simulink model "plant2MRUEBF3_max12"  (R2023b)
settings: Solver=VariableStepAuto  StartTime=0.0  StopTime=7  RelTol=1e-3
model workspace (MATLAB code in the model file):
  | %% Paramètres du Système
  | % Masses
  | mw=0.06;
  | mb=0.894;
  | Ms=mb + 2*mw;
  | 
  | % Distances
  | rho=0.036;
  | l=0.165;
  | d=0.086; % distance A-C
  | 
  | % Electriques
  | L=2.3e-3;
  | R=2.2;
  | % r;
  | 
  | % Couples
  | k=0.347;
  | % alpha=33.5;
  | % beta=2.26e-2;
  | 
  | % Moments inertie A TROUVER
  | Iwy=1.6e-4;
  | Ipsi=3.12e-2;
  | 
  | % Constantes utilitaires
  | beta = (Ms + 2*Iwy/rho^2);
  | gamma = Ipsi + mb*d^2;
  | alpha = 2/rho;
  | eta = l/rho;
  | 
  | % Largeur SensorBar
  | dCLF = 0.09;
  | 
  | %% Trajectoire d'équilibre
  | % Mouvement Rectiligne Uniforme selon axe x du laboratoire.
  | % On néglige les perturbations sur les entrées et les mesures.
  | 
  | % Références
  | ur = 0.3; %m/s
  | psir = 0;
  | 
  | % On fait le changement right,left (r,l) -> sum,dif (s,d)
  | % Somme des tensions gauche et droite
  | % Le "s" signifie "sum", on trouvera aussi "d"
  | % pour "difference"
  | Usbar = 2*k/rho*ur; % should not be >12V
  | Udbar = 0;
  | 
  | Urbar = Usbar/2;
  | Ulbar = Usbar/2;
  | 
  | pbar = 0; % normally, should equals ubar*t,
  | % but is not in state function, so any value fits.
  | ubar = ur;
  | psibar = psir;
  | vbar = 0;
  | Isbar = 0;
  | Idbar = 0;
  | ybar = 0;
  | 
  | statebar = [pbar; ubar; psibar; vbar; Isbar; Idbar; ybar];
  | 
  | %% Sous-système Lent Somme
  | % On a négligé Is par perturbation
  | % Etat=[p; u], Entrée=[Us], Sortie mesurée=[phis]
  | 
  | Qs = k/beta/rho/R;
  | 
  | ASum = [0 1;
  |     0 Qs*(-2*k/rho)];
  | 
  | BSum = [0;
  |     Qs];
  | 
  | CSum = [alpha 0];
  | 
  | DSum = [0];
  | 
  | sysSum = augstate(ss(ASum,BSum,CSum,DSum)); % Ajout de l'état à la sortie
  | set(sysSum,'InputName',{'dUs'},'OutputName',{'dphis','dp','du'});
  | 
  | %% Sous-système Lent Différence
  | % On a négligé Id par perturbation
  | % Etat=[psi; v; y], Entrée=[Ud], Sortie mesurée=[phid; cLF]
  | 
  | b1 = 1/gamma*mb*d*ubar;
  | b2 = 1/gamma*l*k/2/rho/R;
  | 
  | ADif = [0 1 0;
  |     0 (b1 + b2*(-k*l/rho)) 0;
  |     ubar 0 0];
  | 
  | BDif = [0;
  |     b2;
  |     0];
  | 
  | CDif = [eta 0 0;
  |     0 0 1];
  | 
  | DDif = [0;
  |     0];
  | 
  | sysDif = augstate(ss(ADif,BDif,CDif,DDif)); % Ajout de l'état à la sortie
  | set(sysDif,'InputName',{'dUd'},'OutputName',{'dphid','dcLF','dpsi','dv', ...
  |     'dy'});
  | 
  | %% Contrôleurs
  | 
  | %% Modèle de commande somme
  | % réglage PD idéal
  | sumEig = sort(eig(ASum));
  | w0 = 1*abs(sumEig(1)); % accélération facteur 2000
  | xi = 1/sqrt(2);
  | % Gains
  | h1 = w0^2/Qs/alpha;
  | h2 = 1/alpha*(-2*xi*w0/Qs + 2*k/rho);
  | h3 = h1;
  | 
  | % PD approximé
  | Tds = h2/h1;
  | ns = 150; % à régler, augmente la sensibilité au bruit.
  | 
  | 
  | %% Modèle de commande diff
  | 
  | % réglage Contrôleur Idéal, PD sur phid, P sur cLF
  | sigma = 15; % à régler, réponse très lente.
  | % Gains
  | k1 = 1/b2/eta*sigma^2*sqrt(6);
  | k2 = 1/b2/eta*(-sigma*sqrt(6) - b1 + b2*k*l/rho);
  | k3 = k1;
  | k4 = sigma^3/ubar/b2;
  | k5 = k4;
  | difEigDesired = roots([1 sigma*sqrt(6) sigma^2*sqrt(6) sigma^3]);
  | 
  | % PD+D idéal
  | PDdif = [tf([-k2 k3],1) tf([k5],1) tf([k2 -k1],1) tf([-k4],1)];
  | 
  | % PD+P approximé
  | Tdd = k2/k1;
  | nd = 150;
  | 
  | Md = -nd;
  | Nd = [nd 0 -nd 0];
  | Pd = k1*Tdd*nd;
  | Qd = [k1*(1-Tdd*nd) k5 -k1*(1-Tdd*nd) -k5];
  | 
  | %% Etat initial perturbé pour test en poursuite
  | 
  | delta_y = 0.03;
  | delta_psi = pi/2;
  | statebar_perturb = [pbar; ubar; psibar; vbar; Isbar; Idbar; ybar + delta_y];
settings Model: Creator=Jules  LastModifiedBy=Jules

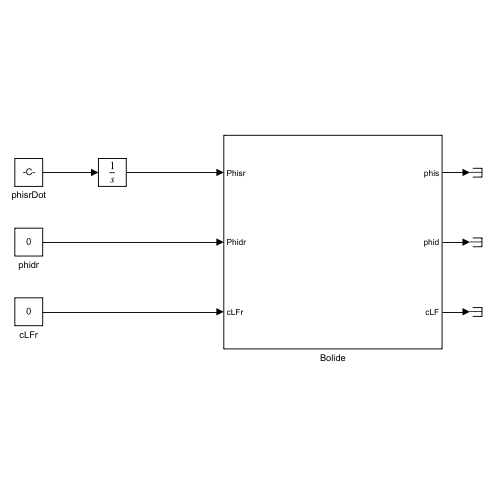
[thumbnail: Simulink's stored preview of the top-level diagram]
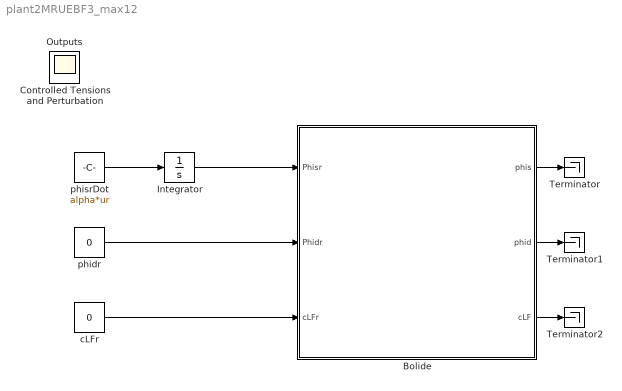
== system plant2MRUEBF3_max12 ==
  Bolide : Subsystem
  Integrator : Integrator
  Terminator : Terminator
  Terminator1 : Terminator
  Terminator2 : Terminator
  cLFr : Constant  Value=0
  phidr : Constant  Value=0
  phisrDot : Constant  Value=alpha*ur
  Controlled Tensions and Perturbation : Scope
  Outputs : Scope
  wires:
  Integrator/1 -> Bolide/1(Phisr)
  phisrDot/1 -> Integrator/1
  phidr/1 -> Bolide/2(Phidr)
  cLFr/1 -> Bolide/3(cLFr)
  Bolide/3(cLF) -> Terminator2/1
  Bolide/2(phid) -> Terminator1/1
  Bolide/1(phis) -> Terminator/1

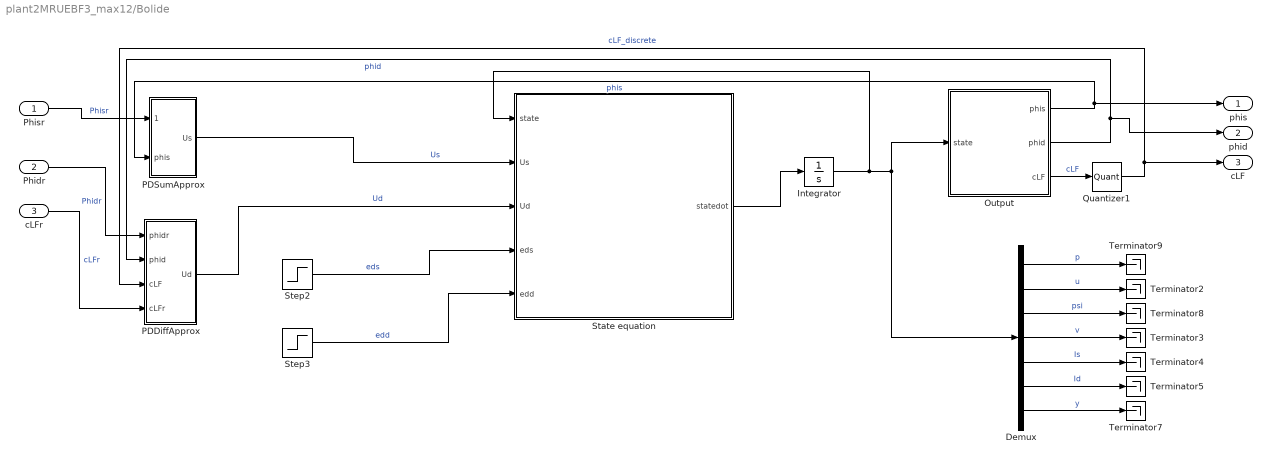
== system plant2MRUEBF3_max12/Bolide ==
  Phisr : Inport
  Phidr : Inport  Port=2
  cLFr : Inport  Port=3
  Demux : Demux  Outputs=7
  Integrator : Integrator  InitialCondition=statebar_perturb
  Output : MATLAB Function  TreatAsAtomicUnit=on
  PDDiffApprox : Subsystem
  PDSumApprox : Subsystem
  Quantizer1 : Quantizer  QuantizationInterval=dCLF/7
  State equation : MATLAB Function  TreatAsAtomicUnit=on
  Step2 : Step  Time=5  After=0  SampleTime=0
  Step3 : Step  Time=2  After=0  SampleTime=0
  Terminator{2..5,7..9} (7 alike) : Terminator
  phis : Outport
  phid : Outport  Port=2
  cLF : Outport  Port=3
  wires:
  Step3/1 -> State equation/5(edd)  "edd"
  State equation/1(statedot) -> Integrator/1
  Step2/1 -> State equation/4(eds)  "eds"
  Demux/1 -> Terminator9/1  "p"
  Demux/7 -> Terminator7/1  "y"
  Demux/2 -> Terminator2/1  "u"
  Demux/6 -> Terminator5/1  "Id"
  Demux/4 -> Terminator3/1  "v"
  Demux/5 -> Terminator4/1  "Is"
  Demux/3 -> Terminator8/1  "psi"
  PDDiffApprox/1(Ud) -> State equation/3(Ud)  "Ud"
  Integrator/1 -> Output/1(state), Demux/1, State equation/1(state)
  Output/1(phis) -> PDSumApprox/2(phis), phis/1  "phis"
  Output/2(phid) -> phid/1, PDDiffApprox/2(phid)  "phid"
  Quantizer1/1 -> PDDiffApprox/3(cLF), cLF/1  "cLF_discrete"
  Phisr/1 -> PDSumApprox/1(phisr)  "Phisr"
  PDSumApprox/1(Us) -> State equation/2(Us)  "Us"
  cLFr/1 -> PDDiffApprox/4(cLFr)  "cLFr"
  Phidr/1 -> PDDiffApprox/1(phidr)  "Phidr"
  Output/3(cLF) -> Quantizer1/1  "cLF"

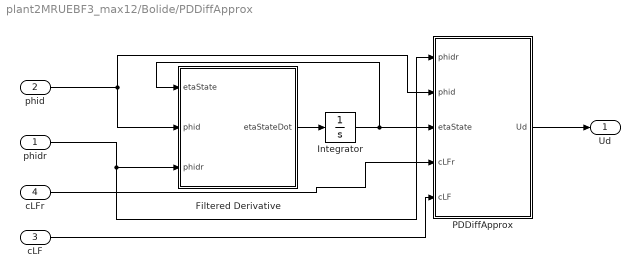
== system plant2MRUEBF3_max12/Bolide/PDDiffApprox ==
  phidr : Inport
  phid : Inport  Port=2
  cLF : Inport  Port=3
  cLFr : Inport  Port=4
  Filtered Derivative : MATLAB Function  TreatAsAtomicUnit=on
  Integrator : Integrator
  PDDiffApprox : MATLAB Function  TreatAsAtomicUnit=on
  Ud : Outport
  wires:
  phidr/1 -> PDDiffApprox/1(phidr), Filtered Derivative/3(phidr)
  phid/1 -> Filtered Derivative/2(phid), PDDiffApprox/2(phid)
  Filtered Derivative/1(etaStateDot) -> Integrator/1
  Integrator/1 -> Filtered Derivative/1(etaState), PDDiffApprox/3(etaState)
  PDDiffApprox/1(Ud) -> Ud/1
  cLF/1 -> PDDiffApprox/5(cLF)
  cLFr/1 -> PDDiffApprox/4(cLFr)

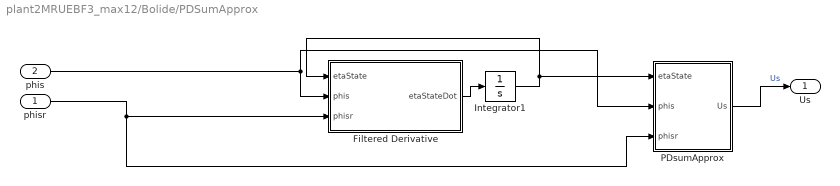
== system plant2MRUEBF3_max12/Bolide/PDSumApprox ==
  phisr : Inport
  phis : Inport  Port=2
  Filtered Derivative : MATLAB Function  TreatAsAtomicUnit=on
  Integrator1 : Integrator
  PDsumApprox : MATLAB Function  TreatAsAtomicUnit=on
  Us : Outport
  wires:
  Integrator1/1 -> Filtered Derivative/1(etaState), PDsumApprox/1(etaState)
  phis/1 -> Filtered Derivative/2(phis), PDsumApprox/2(phis)
  Filtered Derivative/1(etaStateDot) -> Integrator1/1
  phisr/1 -> PDsumApprox/3(phisr), Filtered Derivative/3(phisr)
  PDsumApprox/1(Us) -> Us/1  "Us"

== matlab function plant2MRUEBF3_max12/Bolide/PDSumApprox/Filtered Derivative ==
  data: etaState input; etaStateDot output; phis input; phisr input; ns parameter
function etaStateDot = fcn(etaState,phis,phisr,ns)
deltaPhisr = (phisr - phis);
etaStateDot = ns*(deltaPhisr - etaState);

== matlab function plant2MRUEBF3_max12/Bolide/State equation ==
  data: state input; statedot output; Us input; Ud input; eds input; edd input; beta parameter; gamma parameter; rho parameter; l parameter; d parameter; L parameter; R parameter; k parameter; mb parameter
function statedot = fcn(state, Us, Ud, eds, edd, beta, gamma, rho, l, d, L, R, k, mb)
% ed est l'entrée de perturbation, != d (distance AC)
% Model parameters defined in "Model Explorer/Matlab Code"

p = state(1); % intégrale temporelle de u, distance parcourue
u = state(2);
psi = state(3);
v = state(4); % psidot
Is = state(5); % Intensité à gauche
Id = state(6);
y = state(7); % abscisse point A

% Cap tensions
Ur = 0.5*(Us + Ud);
Ul = 0.5*(Us - Ud);
Ur = max(12.0, Ur);
Ul = max(12.0, Ul);
Us = Ur + Ul;
Ud = Ur - Ul;

pdot = u;
udot = 1/beta*(k/rho*Is - mb*d*v^2);
psidot = v;
vdot = 1/gamma*(l*k/(2*rho)*Id + mb*d*u*v);
Isdot = 1/L*((Us + eds) - R*Is - 2*k/rho*u);
Iddot = 1/L*((Ud + edd) - R*Id - k*l/rho*v);
ydot = sin(psi)*u;

statedot = [pdot; udot; psidot; vdot; Isdot; Iddot; ydot];

== matlab function plant2MRUEBF3_max12/Bolide/PDSumApprox/PDsumApprox ==
  data: etaState input; Us output; phis input; phisr input; h1 parameter; Tds parameter; ns parameter; Usbar parameter
function Us = fcn(etaState,phis,phisr,h1,Tds,ns,Usbar)
deltaPhis = phisr - phis;
Us = Usbar + h1*(1 - Tds*ns)*deltaPhis + h1*Tds*ns*etaState;

== matlab function plant2MRUEBF3_max12/Bolide/Output ==
  data: state input; alpha parameter; phis output; phid output; cLF output; eta parameter
function [phis, phid, cLF] = fcn(state,alpha,eta)
% Sorties mesurées

p = state(1);
psi = state(3);
y = state(7);

phis = alpha*p;
phid = eta*psi;
cLF = y;

== matlab function plant2MRUEBF3_max12/Bolide/PDDiffApprox/Filtered Derivative ==
  data: etaState input; etaStateDot output; phid input; phidr input; nd parameter
function etaStateDot = fcn(etaState,phid,phidr,nd)
deltaPhid = (phidr - phid);
etaStateDot = nd*(deltaPhid - etaState);

== matlab function plant2MRUEBF3_max12/Bolide/PDDiffApprox/PDDiffApprox ==
  data: nd parameter; phidr input; phid input; etaState input; Ud output; cLFr input; cLF input; k1 parameter; k5 parameter; Tdd parameter; Udbar parameter
function Ud = fcn(nd,phidr,phid,etaState,cLFr,cLF,k1,k5,Tdd,Udbar)
deltaPhid = phidr - phid;
deltaCLF = cLFr - cLF;
Ud = Udbar + k1*(1 - Tdd*nd)*deltaPhid + k1*Tdd*nd*etaState + k5*deltaCLF;
